simulink model "quad_1_ref_NN_ports_cex"  (R2018b)
settings: Solver=FixedStepAuto  StartTime=0.0  StopTime=20  FixedStep=0.01  RelTol=1e-3
libraries: neural x348, simulink x2
(part 7 of 13)

== system quad_1_ref_NN_ports_cex/nn_1_const/Layer 3/Delays 1 ==
  "p{3}" : Inport  PortDimensions=30
      mask Display: e = 0.06;c1 = [120 230 180]/255;c2 = ([120 230 180]+0)/(256+128);c3 = ([120 230 180]+128)/(256+128);patch([0 1 1 0],[0 0 1 1],c1);patch([0 1 1 1-e 1-e 0+e],[0 0 1 1-e 0+e 0+e],c2);patch([0 0 1 1-e 0+e 0+e],[0 1 1 1-e 1-e 0+e],c3);plot([0 1 1 0 0],[0 0 1 1 0]);
  mux : Mux  Inputs=1
      mask Display: e = 0.06;c1 = [120 150 230]/255;c2 = ([120 150 230]+0)/383;c3 = ([120 150 230]+128)/383;patch([0 1 1 0],[0 0 1 1],c1);patch([0 1 1 1-e 1-e 0+e],[0 0 1 1-e 0+e 0+e],c2);patch([0 0 1 1-e 0+e 0+e],[0 1 1 1-e 1-e 0+e],c3);plot([0 1 1 0 0],[0 0 1 1 0]);disp('Mux')
  "pd{3,2}" : Outport
      mask Display: e = 0.06;c1 = [120 230 180]/255;c2 = ([120 230 180]+0)/(256+128);c3 = ([120 230 180]+128)/(256+128);patch([0 1 1 0],[0 0 1 1],c1);patch([0 1 1 1-e 1-e 0+e],[0 0 1 1-e 0+e 0+e],c2);patch([0 0 1 1-e 0+e 0+e],[0 1 1 1-e 1-e 0+e],c3);plot([0 1 1 0 0],[0 0 1 1 0]);
  wires:
  "p{3}"/1 -> mux/1
  mux/1 -> "pd{3,2}"/1

== system quad_1_ref_NN_ports_cex/nn_1_const/Layer 3/LW{3,2} ==
  "ad{3,2}" : Inport  PortDimensions=30
      mask Display: e = 0.06;c1 = [120 230 180]/255;c2 = ([120 230 180]+0)/(256+128);c3 = ([120 230 180]+128)/(256+128);patch([0 1 1 0],[0 0 1 1],c1);patch([0 1 1 1-e 1-e 0+e],[0 0 1 1-e 0+e 0+e],c2);patch([0 0 1 1-e 0+e 0+e],[0 1 1 1-e 1-e 0+e],c3);plot([0 1 1 0 0],[0 0 1 1 0]);
  "IW{3,2}(1,:)'" : Constant  Value=[0.327928758624340732641400109059759415686130523681640625;-0.55820440747247535018260577999171800911426544189453125;-0.271204192099869789700505862128920853137969970703125;-0.0557769100753577884432843347894959151744842529296875;-0.32758772482643194745577375215361826121807098388671875;0.0203657576424367860179476252824315452016890048980712890625;0.07347277676480434838168775968370027840137481689453125;-0.1579526322944761196342966513839201070368289947509765625;-0.325542754449849980336040289330412633717060089111328125;-0.2238280397863224580046193068483262322843074798583984375;-0.320888627943421378407862221138202585279941558837890625;-0.1946744660874496213320838933213963173329830169677734375;0.50023714377249006712844447974930517375469207763671875;0.1229991088401860277468102822240325622260570526123046875;0.23866675410597848472349369330913759768009185791015625;-0.108125456895287130887339799301116727292537689208984375;-0.491825485074962320819480510181165300309658050537109375;-0.038901938867322134740778238892744411714375019073486328125;0.1040818180648106772157035493364674039185047149658203125;-0.376891881907984116484300329830148257315158843994140625;0.0994428292402699531837839685977087356150150299072265625;-0.07984307261712157710586978964784066192805767059326171875;-0.50048749643499268469071239451295696198940277099609375;-0.45905895663722462440858862464665435254573822021484375;-0.352625950373064878107243202975951135158538818359375;0.1980733704162148944849519693889305926859378814697265625;0.34322332885967565818674529509735293686389923095703125;0.307778286204612172571870587489684112370014190673828125;0.1738835713025933260578170802546082995831966400146484375;-0.23217221679979294091111796660698018968105316162109375]
      mask Display: e = 0.06;c1 = [120 150 230]/255;c2 = ([120 150 230]+0)/383;c3 = ([120 150 230]+128)/383;patch([0 1 1 0],[0 0 1 1],c1);patch([0 1 1 1-e 1-e 0+e],[0 0 1 1-e 0+e 0+e],c2);patch([0 0 1 1-e 0+e 0+e],[0 1 1 1-e 1-e 0+e],c3);plot([0 1 1 0 0],[0 0 1 1 0]);disp('weights');
  "IW{3,2}(2,:)'" : Constant  Value=[-0.10809198337702830006179510746733285486698150634765625;0.1269626329970421074744280076629365794360637664794921875;-0.04521852435502367317798899648551014252007007598876953125;0.1503614425428999312739364313529222272336483001708984375;-0.34833058785911663601808641033130697906017303466796875;0.27979681620865737290415609095362015068531036376953125;-0.3819593294524763482655771440477110445499420166015625;-0.412433724296779657958467169009963981807231903076171875;0.3315789715870411935583206286537460982799530029296875;-0.05820866646834126079124160924038733355700969696044921875;0.306906948135961477053257340230629779398441314697265625;0.37252585636531143631344775712932460010051727294921875;0.308636286795391512338682105109910480678081512451171875;0.2246537489971980050551536578495870344340801239013671875;-0.319882615763760480565025545729440636932849884033203125;-0.00488583502039973728570121380698765278793871402740478515625;0.150436498090291859153211362354340963065624237060546875;0.345641424157331955679950397097854875028133392333984375;0.2227838823473465013069727547190268523991107940673828125;-0.35474970617276746498447437261347658932209014892578125;-0.161697319640236758520046578269102610647678375244140625;-0.44222403234847507125238053049542941153049468994140625;0.211200082911826181319980832995497621595859527587890625;0.42181878561118490988945950448396615684032440185546875;0.03042048915592758528969596909519168548285961151123046875;-0.1897801641563659769129657206576666794717311859130859375;0.1173103045554617918089235217848909087479114532470703125;-0.39376723264394986045999758061952888965606689453125;-0.3681839900591972192245293626911006867885589599609375;0.24280439564999445334336769519723020493984222412109375]
      mask Display: e = 0.06;c1 = [120 150 230]/255;c2 = ([120 150 230]+0)/383;c3 = ([120 150 230]+128)/383;patch([0 1 1 0],[0 0 1 1],c1);patch([0 1 1 1-e 1-e 0+e],[0 0 1 1-e 0+e 0+e],c2);patch([0 0 1 1-e 0+e 0+e],[0 1 1 1-e 1-e 0+e],c3);plot([0 1 1 0 0],[0 0 1 1 0]);disp('weights');
  "IW{3,2}(3,:)'" : Constant  Value=[-0.09740648016186574664754260766130755655467510223388671875;0.1464692614288338745609507896006107330322265625;0.1236987666034225219480191526599810458719730377197265625;0.2380814753048181575678654553485102951526641845703125;0.2303349187376148854422552858522976748645305633544921875;-0.351436586776914750007705379175604321062564849853515625;-0.355839979865836320005456627768580801784992218017578125;-0.12645189201681328317050656551145948469638824462890625;-0.360175944289336913417542973547824658453464508056640625;-0.44453119511866912016984088040771894156932830810546875;0.193836852370338819095962890060036443173885345458984375;0.17499175809764644373700548385386355221271514892578125;0.34285036708253080472985629967297427356243133544921875;-0.28300354963433915767012649666867218911647796630859375;-0.182825795105293231745946513910894282162189483642578125;0.01097749415561990148082482932068160152994096279144287109375;0.38174355853860764131724181424942798912525177001953125;-0.31918936839138634109502845603856258094310760498046875;-0.37820437326661970889318808985990472137928009033203125;0.395234944564560597424218713058508001267910003662109375;0.462073063934263672525304400551249273121356964111328125;-0.31942243334065911763985923244035802781581878662109375;0.415880057336451447458358643416431732475757598876953125;-0.29086088149263644719866306331823579967021942138671875;0.394363290651797926411603611995815299451351165771484375;0.3847585799648449711440889586810953915119171142578125;-0.319785572536297302281838028648053295910358428955078125;0.4503165790658680833757898653857409954071044921875;-0.2488760245881067867390612491362844593822956085205078125;0.231892196915004900059642523046932183206081390380859375]
      mask Display: e = 0.06;c1 = [120 150 230]/255;c2 = ([120 150 230]+0)/383;c3 = ([120 150 230]+128)/383;patch([0 1 1 0],[0 0 1 1],c1);patch([0 1 1 1-e 1-e 0+e],[0 0 1 1-e 0+e 0+e],c2);patch([0 0 1 1-e 0+e 0+e],[0 1 1 1-e 1-e 0+e],c3);plot([0 1 1 0 0],[0 0 1 1 0]);disp('weights');
  Mux : Mux  Inputs=3
      mask Display: e = 0.06;c1 = [120 150 230]/255;c2 = ([120 150 230]+0)/383;c3 = ([120 150 230]+128)/383;patch([0 1 1 0],[0 0 1 1],c1);patch([0 1 1 1-e 1-e 0+e],[0 0 1 1-e 0+e 0+e],c2);patch([0 0 1 1-e 0+e 0+e],[0 1 1 1-e 1-e 0+e],c3);plot([0 1 1 0 0],[0 0 1 1 0]);disp('Mux');
  dotprod1 : neural/Weight Functions/dotprod
  dotprod2 : neural/Weight Functions/dotprod
  dotprod3 : neural/Weight Functions/dotprod
  "lz{3,2}" : Outport
      mask Display: e = 0.06;c1 = [120 230 180]/255;c2 = ([120 230 180]+0)/(256+128);c3 = ([120 230 180]+128)/(256+128);patch([0 1 1 0],[0 0 1 1],c1);patch([0 1 1 1-e 1-e 0+e],[0 0 1 1-e 0+e 0+e],c2);patch([0 0 1 1-e 0+e 0+e],[0 1 1 1-e 1-e 0+e],c3);plot([0 1 1 0 0],[0 0 1 1 0]);
  wires:
  "IW{3,2}(1,:)'"/1 -> dotprod1/1
  "ad{3,2}"/1 -> dotprod1/2, dotprod2/2, dotprod3/2
  dotprod1/1 -> Mux/1
  "IW{3,2}(2,:)'"/1 -> dotprod2/1
  dotprod2/1 -> Mux/2
  "IW{3,2}(3,:)'"/1 -> dotprod3/1
  dotprod3/1 -> Mux/3
  Mux/1 -> "lz{3,2}"/1

== system quad_1_ref_NN_ports_cex/nn_2/Layer 1/Delays 1 ==
  "p{1}" : Inport  PortDimensions=12
      mask Display: e = 0.06;c1 = [120 230 180]/255;c2 = ([120 230 180]+0)/(256+128);c3 = ([120 230 180]+128)/(256+128);patch([0 1 1 0],[0 0 1 1],c1);patch([0 1 1 1-e 1-e 0+e],[0 0 1 1-e 0+e 0+e],c2);patch([0 0 1 1-e 0+e 0+e],[0 1 1 1-e 1-e 0+e],c3);plot([0 1 1 0 0],[0 0 1 1 0]);
  mux : Mux  Inputs=1
      mask Display: e = 0.06;c1 = [120 150 230]/255;c2 = ([120 150 230]+0)/383;c3 = ([120 150 230]+128)/383;patch([0 1 1 0],[0 0 1 1],c1);patch([0 1 1 1-e 1-e 0+e],[0 0 1 1-e 0+e 0+e],c2);patch([0 0 1 1-e 0+e 0+e],[0 1 1 1-e 1-e 0+e],c3);plot([0 1 1 0 0],[0 0 1 1 0]);disp('Mux')
  "pd{1,1}" : Outport
      mask Display: e = 0.06;c1 = [120 230 180]/255;c2 = ([120 230 180]+0)/(256+128);c3 = ([120 230 180]+128)/(256+128);patch([0 1 1 0],[0 0 1 1],c1);patch([0 1 1 1-e 1-e 0+e],[0 0 1 1-e 0+e 0+e],c2);patch([0 0 1 1-e 0+e 0+e],[0 1 1 1-e 1-e 0+e],c3);plot([0 1 1 0 0],[0 0 1 1 0]);
  wires:
  "p{1}"/1 -> mux/1
  mux/1 -> "pd{1,1}"/1

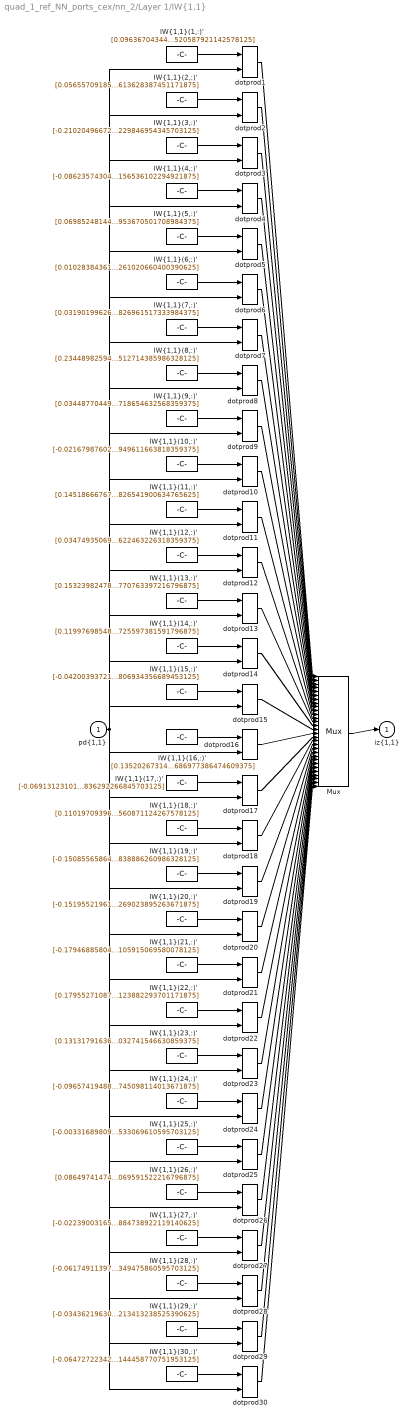
== system quad_1_ref_NN_ports_cex/nn_2/Layer 1/IW{1,1} ==
  "pd{1,1}" : Inport  PortDimensions=12
      mask Display: e = 0.06;c1 = [120 230 180]/255;c2 = ([120 230 180]+0)/(256+128);c3 = ([120 230 180]+128)/(256+128);patch([0 1 1 0],[0 0 1 1],c1);patch([0 1 1 1-e 1-e 0+e],[0 0 1 1-e 0+e 0+e],c2);patch([0 0 1 1-e 0+e 0+e],[0 1 1 1-e 1-e 0+e],c3);plot([0 1 1 0 0],[0 0 1 1 0]);
  "IW{1,1}(1,:)'" : Constant  Value=[0.0963670434492417127270158516694209538400173187255859375;-0.02998489557824503271010740945712313987314701080322265625;0.0198357262796998133624892801663008867762982845306396484375;-0.233494818149912131133305592811666429042816162109375;-0.03964733773014815498836327378739952109754085540771484375;-0.055871328120397911742855967531795613467693328857421875;0.10744492173777138444012990703413379378616809844970703125;-0.0132970271938564719993447482693227357231080532073974609375;0.04911326928811628189652793707864475436508655548095703125;0.03458487107728924758731636757147498428821563720703125;-0.0359117782994806955532141046205651946365833282470703125;0.033230187979102217277205255641092662699520587921142578125]
      mask Display: e = 0.06;c1 = [120 150 230]/255;c2 = ([120 150 230]+0)/383;c3 = ([120 150 230]+128)/383;patch([0 1 1 0],[0 0 1 1],c1);patch([0 1 1 1-e 1-e 0+e],[0 0 1 1-e 0+e 0+e],c2);patch([0 0 1 1-e 0+e 0+e],[0 1 1 1-e 1-e 0+e],c3);plot([0 1 1 0 0],[0 0 1 1 0]);disp('Weights');
  "IW{1,1}(10,:)'" : Constant  Value=[-0.02167987602032135641128007819133927114307880401611328125;0.009575603101159756158633484801612212322652339935302734375;0.06250670535464737664899104174764943309128284454345703125;-0.090538462652213380632559847072116099298000335693359375;0.07271725243563265106416793059906922280788421630859375;-0.0789953395984055728451522782052052207291126251220703125;0.01895637010247945564156424325119587592780590057373046875;-0.02135735691323818741249596087072859518229961395263671875;0.038366841864127775030279821066869772039353847503662109375;0.02384723046277258118319508639615378342568874359130859375;-0.057235972875386113833950929574712063185870647430419921875;0.0258863878959363601095500229121171287260949611663818359375]
      mask Display: e = 0.06;c1 = [120 150 230]/255;c2 = ([120 150 230]+0)/383;c3 = ([120 150 230]+128)/383;patch([0 1 1 0],[0 0 1 1],c1);patch([0 1 1 1-e 1-e 0+e],[0 0 1 1-e 0+e 0+e],c2);patch([0 0 1 1-e 0+e 0+e],[0 1 1 1-e 1-e 0+e],c3);plot([0 1 1 0 0],[0 0 1 1 0]);disp('Weights');
  "IW{1,1}(11,:)'" : Constant  Value=[0.145186667677384750874125529662705957889556884765625;-0.0207530656856331485737854336548480205237865447998046875;-0.066554745131548964653944722158485092222690582275390625;-0.1590044911041626207737209597326000221073627471923828125;-0.0487637284564807760300908512363093905150890350341796875;0.048655868081689403192857668045689933933317661285400390625;0.07936960987217712981678374717375845648348331451416015625;0.0304471844088852160170599603361551999114453792572021484375;0.0237727270256750493337971619212112273089587688446044921875;0.0240198276716949744857831916533541516400873661041259765625;-0.02189528829818498945058991012047044932842254638671875;-0.032706422447001094744312155171428457833826541900634765625]
      mask Display: e = 0.06;c1 = [120 150 230]/255;c2 = ([120 150 230]+0)/383;c3 = ([120 150 230]+128)/383;patch([0 1 1 0],[0 0 1 1],c1);patch([0 1 1 1-e 1-e 0+e],[0 0 1 1-e 0+e 0+e],c2);patch([0 0 1 1-e 0+e 0+e],[0 1 1 1-e 1-e 0+e],c3);plot([0 1 1 0 0],[0 0 1 1 0]);disp('Weights');
  "IW{1,1}(12,:)'" : Constant  Value=[0.034749350696773102786796272312130895443260669708251953125;-0.0736014333872269388425735314740450121462345123291015625;-0.037388165088897341858942269254839629866182804107666015625;0.04756893471249269700340533972848788835108280181884765625;-0.10311435477450504871743675039397203363478183746337890625;0.11262509738201705034033039964924682863056659698486328125;0.0272244869768578333368846955409026122651994228363037109375;-0.018690262067379316557325097392094903625547885894775390625;0.01411732975557855769566106829415730317123234272003173828125;-0.08312468015204542426399569876593886874616146087646484375;-0.052782509266411987980394115993476589210331439971923828125;0.0021418031183407320282297003899429910234175622463226318359375]
      mask Display: e = 0.06;c1 = [120 150 230]/255;c2 = ([120 150 230]+0)/383;c3 = ([120 150 230]+128)/383;patch([0 1 1 0],[0 0 1 1],c1);patch([0 1 1 1-e 1-e 0+e],[0 0 1 1-e 0+e 0+e],c2);patch([0 0 1 1-e 0+e 0+e],[0 1 1 1-e 1-e 0+e],c3);plot([0 1 1 0 0],[0 0 1 1 0]);disp('Weights');
  "IW{1,1}(13,:)'" : Constant  Value=[0.1532398247813539782224978580416063778102397918701171875;0.06953247036407035619465233367009204812347888946533203125;0.00514430221877268216423839675144336069934070110321044921875;-0.171861418147732425421025936884689144790172576904296875;0.046461345556491291663991916038867202587425708770751953125;-0.041708795666123420209370209477128810249269008636474609375;0.041362902434634689352588310384817305020987987518310546875;-0.059449582565483972962372405390851781703531742095947265625;0.0097410876172814020446111271667177788913249969482421875;0.01049776314909686529552867995107590104453265666961669921875;0.033633962417937750266627716655420954339206218719482421875;0.03356606858325654474395349780024844221770763397216796875]
      mask Display: e = 0.06;c1 = [120 150 230]/255;c2 = ([120 150 230]+0)/383;c3 = ([120 150 230]+128)/383;patch([0 1 1 0],[0 0 1 1],c1);patch([0 1 1 1-e 1-e 0+e],[0 0 1 1-e 0+e 0+e],c2);patch([0 0 1 1-e 0+e 0+e],[0 1 1 1-e 1-e 0+e],c3);plot([0 1 1 0 0],[0 0 1 1 0]);disp('Weights');
  "IW{1,1}(14,:)'" : Constant  Value=[0.119976985486957066218138834301498718559741973876953125;0.011074455843699294865789539699107990600168704986572265625;-0.005488285907870558109900027687899637385271489620208740234375;-0.26835186485985718096713981140055693686008453369140625;-0.054938731032241512608482736368387122638523578643798828125;0.0149095357482565936402263417903668596409261226654052734375;0.1518363114705344185662028166916570626199245452880859375;0.027439598095624843920870006286349962465465068817138671875;0.01067608020442331086263809680758640752173960208892822265625;-0.043888814704480368089622999150378745980560779571533203125;0.017947586174126069213929923762407270260155200958251953125;-0.00965387200216295641996833154507839935831725597381591796875]
      mask Display: e = 0.06;c1 = [120 150 230]/255;c2 = ([120 150 230]+0)/383;c3 = ([120 150 230]+128)/383;patch([0 1 1 0],[0 0 1 1],c1);patch([0 1 1 1-e 1-e 0+e],[0 0 1 1-e 0+e 0+e],c2);patch([0 0 1 1-e 0+e 0+e],[0 1 1 1-e 1-e 0+e],c3);plot([0 1 1 0 0],[0 0 1 1 0]);disp('Weights');
  "IW{1,1}(15,:)'" : Constant  Value=[-0.0420039372100648733532324285988579504191875457763671875;-0.002762984426971562719466124491418668185360729694366455078125;0.009128102130523889357061051441633026115596294403076171875;-0.14647320652433093446376233259798027575016021728515625;0.046914158427741624313167534410240477882325649261474609375;-0.0277928987001266648848574192243177094496786594390869140625;-0.054667118131341237152742706939534400589764118194580078125;-0.0251059154922964877787450177493155933916568756103515625;-0.07223823520848195178789552528542117215692996978759765625;-0.0167336904534491660856421191283516236580908298492431640625;0.04191004740064542544164538639961392618715763092041015625;-0.051084165943738442383637021748654660768806934356689453125]
      mask Display: e = 0.06;c1 = [120 150 230]/255;c2 = ([120 150 230]+0)/383;c3 = ([120 150 230]+128)/383;patch([0 1 1 0],[0 0 1 1],c1);patch([0 1 1 1-e 1-e 0+e],[0 0 1 1-e 0+e 0+e],c2);patch([0 0 1 1-e 0+e 0+e],[0 1 1 1-e 1-e 0+e],c3);plot([0 1 1 0 0],[0 0 1 1 0]);disp('Weights');
  "IW{1,1}(16,:)'" : Constant  Value=[0.1352026731469619935666059973300434648990631103515625;-0.047386257163045071572060606968079810030758380889892578125;-0.041907967250772427958427357452819705940783023834228515625;-0.1563236402964026383610729453721432946622371673583984375;-0.0235850694502852016587457484320111689157783985137939453125;0.0116247438816773455971809170250708120875060558319091796875;-0.040658251599097562645201975328745902515947818756103515625;0.05251236963362911069896910021270741708576679229736328125;-0.01102946874268842698818549052930393372662365436553955078125;-0.005492271286121085116516127300201333127915859222412109375;0.0234165142870034724553729432727777748368680477142333984375;-0.040401643285461863452923125805682502686977386474609375]
      mask Display: e = 0.06;c1 = [120 150 230]/255;c2 = ([120 150 230]+0)/383;c3 = ([120 150 230]+128)/383;patch([0 1 1 0],[0 0 1 1],c1);patch([0 1 1 1-e 1-e 0+e],[0 0 1 1-e 0+e 0+e],c2);patch([0 0 1 1-e 0+e 0+e],[0 1 1 1-e 1-e 0+e],c3);plot([0 1 1 0 0],[0 0 1 1 0]);disp('Weights');
  "IW{1,1}(17,:)'" : Constant  Value=[-0.06913123101193986708157268594732158817350864410400390625;-0.042455432406210295848136837548736366443336009979248046875;0.01369205857005208193388767767828539945185184478759765625;0.11383782048737491054968273829217650927603244781494140625;-0.060466490543143340541387686926100286655128002166748046875;0.0188919876523014375335751680040630162693560123443603515625;-0.048107408169124142582884218199978931806981563568115234375;-0.01528739302378535717952257044771613436751067638397216796875;-0.05144260921280367770958008577508735470473766326904296875;-0.05096443422523273814039868057079729624092578887939453125;-0.02945636339152606086866370560528594069182872772216796875;-0.0171135307590550740652890482351722312159836292266845703125]
      mask Display: e = 0.06;c1 = [120 150 230]/255;c2 = ([120 150 230]+0)/383;c3 = ([120 150 230]+128)/383;patch([0 1 1 0],[0 0 1 1],c1);patch([0 1 1 1-e 1-e 0+e],[0 0 1 1-e 0+e 0+e],c2);patch([0 0 1 1-e 0+e 0+e],[0 1 1 1-e 1-e 0+e],c3);plot([0 1 1 0 0],[0 0 1 1 0]);disp('Weights');
  "IW{1,1}(18,:)'" : Constant  Value=[0.11019709396075240415147078465452068485319614410400390625;0.04926979088195641842684580069544608704745769500732421875;-0.04838283233660277404819538560332148335874080657958984375;-0.00963057704813059800574848168253083713352680206298828125;-0.009613748734012779462165809718499076552689075469970703125;-0.0325377541810061010618682075801189057528972625732421875;0.036575137550091195437484969943398027680814266204833984375;-0.01572076232144341279006738432144629769027233123779296875;-0.0076129085484086013446702878582073026336729526519775390625;-0.025254150868068779567376935801803483627736568450927734375;-0.046262519846408341195331814788005431182682514190673828125;-0.040657774038491974188946898038921062834560871124267578125]
      mask Display: e = 0.06;c1 = [120 150 230]/255;c2 = ([120 150 230]+0)/383;c3 = ([120 150 230]+128)/383;patch([0 1 1 0],[0 0 1 1],c1);patch([0 1 1 1-e 1-e 0+e],[0 0 1 1-e 0+e 0+e],c2);patch([0 0 1 1-e 0+e 0+e],[0 1 1 1-e 1-e 0+e],c3);plot([0 1 1 0 0],[0 0 1 1 0]);disp('Weights');
  "IW{1,1}(19,:)'" : Constant  Value=[-0.1508556586474403271580513319349847733974456787109375;-0.018213648918746681848457313890321529470384120941162109375;-0.027881145100316861995537465190864168107509613037109375;0.1829520964826169826533686091352137736976146697998046875;-0.048285945392414646171186376477635349147021770477294921875;0.054448955430182501002978057158543379046022891998291015625;-0.10379420330937040584107222684906446374952793121337890625;0.019158116711153423683544616551444050855934619903564453125;0.039685064615922575892437151878766599111258983612060546875;-0.0231794568681364422657598112209598184563219547271728515625;0.0055987528789933523054589414869042229838669300079345703125;-0.016475006097132767479696013879220117814838886260986328125]
      mask Display: e = 0.06;c1 = [120 150 230]/255;c2 = ([120 150 230]+0)/383;c3 = ([120 150 230]+128)/383;patch([0 1 1 0],[0 0 1 1],c1);patch([0 1 1 1-e 1-e 0+e],[0 0 1 1-e 0+e 0+e],c2);patch([0 0 1 1-e 0+e 0+e],[0 1 1 1-e 1-e 0+e],c3);plot([0 1 1 0 0],[0 0 1 1 0]);disp('Weights');
  "IW{1,1}(2,:)'" : Constant  Value=[0.0565570918586223714275007523610838688910007476806640625;-0.04556319233391274703404150159258279018104076385498046875;-0.00525403129053085560240532458919915370643138885498046875;-0.02284769747955449348264522768658935092389583587646484375;-0.043835671970937857555572492174178478308022022247314453125;-0.041265694783639894627214061983977444469928741455078125;-0.0137285514204576741814634033289621584117412567138671875;0.0251722865985351089423982529069689917378127574920654296875;0.041086109140649702820002886483052861876785755157470703125;0.044350373424499579810831306758700520731508731842041015625;0.0297244917886227318082337234272927162237465381622314453125;-0.017723255711821921110082911354766110889613628387451171875]
      mask Display: e = 0.06;c1 = [120 150 230]/255;c2 = ([120 150 230]+0)/383;c3 = ([120 150 230]+128)/383;patch([0 1 1 0],[0 0 1 1],c1);patch([0 1 1 1-e 1-e 0+e],[0 0 1 1-e 0+e 0+e],c2);patch([0 0 1 1-e 0+e 0+e],[0 1 1 1-e 1-e 0+e],c3);plot([0 1 1 0 0],[0 0 1 1 0]);disp('Weights');
  "IW{1,1}(20,:)'" : Constant  Value=[-0.151955219615692527224126706641982309520244598388671875;-0.00644169278533961685295761157021843246184289455413818359375;-0.0014910754802380308918496876202652856591157615184783935546875;0.2178704362857331877645350459715700708329677581787109375;-0.0159318550347393970978426835927166393958032131195068359375;-0.0306780730434982780441277583349801716394722461700439453125;-0.165514568504929793224533796092146076261997222900390625;-0.03816639102354042745179896201079827733337879180908203125;0.048144549460101222770891382651825551874935626983642578125;-0.04926366893596752227768575949085061438381671905517578125;0.00583623873334166744231144008381306775845587253570556640625;-0.038415089615007107226585247872208128683269023895263671875]
      mask Display: e = 0.06;c1 = [120 150 230]/255;c2 = ([120 150 230]+0)/383;c3 = ([120 150 230]+128)/383;patch([0 1 1 0],[0 0 1 1],c1);patch([0 1 1 1-e 1-e 0+e],[0 0 1 1-e 0+e 0+e],c2);patch([0 0 1 1-e 0+e 0+e],[0 1 1 1-e 1-e 0+e],c3);plot([0 1 1 0 0],[0 0 1 1 0]);disp('Weights');
  "IW{1,1}(21,:)'" : Constant  Value=[-0.1794688580443983827450438184314407408237457275390625;-0.028516979645142041810412791846829350106418132781982421875;-0.0090720363478705122461942522704703151248395442962646484375;0.1255159624610372726127849318800144828855991363525390625;-0.039600857039564930917041607472128816880285739898681640625;-0.032308661764052060139107425129623152315616607666015625;-0.016981166020414890927003881415657815523445606231689453125;0.03632720422941571047914521841448731720447540283203125;-0.000448192583532860087947025107268927968107163906097412109375;0.01167939131266501097405896558711901889182627201080322265625;0.054971223698895892162408216563562746159732341766357421875;0.0015702044461439715501704927902437702869065105915069580078125]
      mask Display: e = 0.06;c1 = [120 150 230]/255;c2 = ([120 150 230]+0)/383;c3 = ([120 150 230]+128)/383;patch([0 1 1 0],[0 0 1 1],c1);patch([0 1 1 1-e 1-e 0+e],[0 0 1 1-e 0+e 0+e],c2);patch([0 0 1 1-e 0+e 0+e],[0 1 1 1-e 1-e 0+e],c3);plot([0 1 1 0 0],[0 0 1 1 0]);disp('Weights');
  "IW{1,1}(22,:)'" : Constant  Value=[0.179552710875321486216904531829641200602054595947265625;-0.0271027099443047377047566470764650148339569568634033203125;-0.0668122147617648820538960308113018982112407684326171875;-0.2312456882295024496176694128735107369720935821533203125;-0.0572558162532104952813227782826288603246212005615234375;0.092657437825664545893999957115738652646541595458984375;0.10313999906360561686913257517517195083200931549072265625;-0.0271104480045279705446858997675008140504360198974609375;0.0114841311289845850185376008312232443131506443023681640625;0.030408296426441328019762977419304661452770233154296875;0.0307288869733456648791758425431908108294010162353515625;-0.017814450901100280233446682132125715725123882293701171875]
      mask Display: e = 0.06;c1 = [120 150 230]/255;c2 = ([120 150 230]+0)/383;c3 = ([120 150 230]+128)/383;patch([0 1 1 0],[0 0 1 1],c1);patch([0 1 1 1-e 1-e 0+e],[0 0 1 1-e 0+e 0+e],c2);patch([0 0 1 1-e 0+e 0+e],[0 1 1 1-e 1-e 0+e],c3);plot([0 1 1 0 0],[0 0 1 1 0]);disp('Weights');
  "IW{1,1}(23,:)'" : Constant  Value=[0.13131791636346878959784589824266731739044189453125;0.0193863240459271994609036227075193892233073711395263671875;0.00715174559120907750442430739212795742787420749664306640625;0.05486655159595266173511163287912495434284210205078125;0.0401442208550966406210847026159171946346759796142578125;0.04377915024574856317496340807338128797709941864013671875;-0.031675194504130137207464912307841586880385875701904296875;0.01981077134609214585037051392646390013396739959716796875;-0.00963765867608215066886234723142479197122156620025634765625;-0.047466276118460902500029163775252527557313442230224609375;-0.01166577285425598499435384525213521555997431278228759765625;-0.0197833266932704032736722865593037568032741546630859375]
      mask Display: e = 0.06;c1 = [120 150 230]/255;c2 = ([120 150 230]+0)/383;c3 = ([120 150 230]+128)/383;patch([0 1 1 0],[0 0 1 1],c1);patch([0 1 1 1-e 1-e 0+e],[0 0 1 1-e 0+e 0+e],c2);patch([0 0 1 1-e 0+e 0+e],[0 1 1 1-e 1-e 0+e],c3);plot([0 1 1 0 0],[0 0 1 1 0]);disp('Weights');
  "IW{1,1}(24,:)'" : Constant  Value=[-0.09657419488549467967430928183603100478649139404296875;0.0241557095740239750891742431804232182912528514862060546875;0.047777796487195108021683864762962912209331989288330078125;0.1623879706509529785574130755776423029601573944091796875;-0.0456818379862133083779696107740164734423160552978515625;-0.0200364773549174639277747900223403121344745159149169921875;-0.07744412917817887487270667179473093710839748382568359375;0.020062417659231446265266640693880617618560791015625;-0.061868560782029576039509066731625352986156940460205078125;0.067823465106819968983842272791662253439426422119140625;0.03182642212306575901781258153278031386435031890869140625;0.031288377204634225392521074127216706983745098114013671875]
      mask Display: e = 0.06;c1 = [120 150 230]/255;c2 = ([120 150 230]+0)/383;c3 = ([120 150 230]+128)/383;patch([0 1 1 0],[0 0 1 1],c1);patch([0 1 1 1-e 1-e 0+e],[0 0 1 1-e 0+e 0+e],c2);patch([0 0 1 1-e 0+e 0+e],[0 1 1 1-e 1-e 0+e],c3);plot([0 1 1 0 0],[0 0 1 1 0]);disp('Weights');
  "IW{1,1}(25,:)'" : Constant  Value=[-0.00331689809484806384654032029857262386940419673919677734375;-0.000282766784016928360810660958435391876264475286006927490234375;0.00831186986145609520149069027183941216208040714263916015625;-0.030673501351737054998469744759859167970716953277587890625;-0.043560595315479601341568383077174075879156589508056640625;-0.059214945748563764527094832601505913771688938140869140625;-0.0073905937341639908744195253120778943412005901336669921875;0.051288395431760676335120052726779249496757984161376953125;0.07664423673696525718401773019650136120617389678955078125;0.03814554995943862658602796500417753122746944427490234375;-0.01543352955019334192543478678771862178109586238861083984375;-0.01042068425015845074821374538487361860461533069610595703125]
      mask Display: e = 0.06;c1 = [120 150 230]/255;c2 = ([120 150 230]+0)/383;c3 = ([120 150 230]+128)/383;patch([0 1 1 0],[0 0 1 1],c1);patch([0 1 1 1-e 1-e 0+e],[0 0 1 1-e 0+e 0+e],c2);patch([0 0 1 1-e 0+e 0+e],[0 1 1 1-e 1-e 0+e],c3);plot([0 1 1 0 0],[0 0 1 1 0]);disp('Weights');
  "IW{1,1}(26,:)'" : Constant  Value=[0.0864974147458101028096422169255674816668033599853515625;0.040666463190978892339177974690755945630371570587158203125;0.00946664496001405585123844588224528706632554531097412109375;-0.04383941989612703815648586669340147636830806732177734375;0.03127239447551567741445666115396306850016117095947265625;-0.0157148210500004971434950817865683347918093204498291015625;0.04288729634681824609554467997440951876342296600341796875;0.045272834343532318557290494709377526305615901947021484375;0.002130217585906197912126724958170598256401717662811279296875;-0.039506203531120311078783657876556389965116977691650390625;-0.04856855204270905945751479748651036061346530914306640625;-0.026968614233296654691951488302947836928069591522216796875]
      mask Display: e = 0.06;c1 = [120 150 230]/255;c2 = ([120 150 230]+0)/383;c3 = ([120 150 230]+128)/383;patch([0 1 1 0],[0 0 1 1],c1);patch([0 1 1 1-e 1-e 0+e],[0 0 1 1-e 0+e 0+e],c2);patch([0 0 1 1-e 0+e 0+e],[0 1 1 1-e 1-e 0+e],c3);plot([0 1 1 0 0],[0 0 1 1 0]);disp('Weights');
  "IW{1,1}(27,:)'" : Constant  Value=[-0.02239003165257756611250528067103005014359951019287109375;-0.0538707440898208156365711829494102858006954193115234375;-0.0330754878358191783949138198295258916914463043212890625;-0.035570346482772803586858145763471839018166065216064453125;0.02574992367182293850902397025492973625659942626953125;-0.058123079327492187251547051118905073963105678558349609375;0.060044248722781239091528249218754353933036327362060546875;0.007465947049040411176434872686513699591159820556640625;0.01239835981269137889226872317749439389444887638092041015625;0.0094665618527167323670301612992261652834713459014892578125;0.0226138083092675967744611398302367888391017913818359375;-0.0659262781382616014358433176312246359884738922119140625]
      mask Display: e = 0.06;c1 = [120 150 230]/255;c2 = ([120 150 230]+0)/383;c3 = ([120 150 230]+128)/383;patch([0 1 1 0],[0 0 1 1],c1);patch([0 1 1 1-e 1-e 0+e],[0 0 1 1-e 0+e 0+e],c2);patch([0 0 1 1-e 0+e 0+e],[0 1 1 1-e 1-e 0+e],c3);plot([0 1 1 0 0],[0 0 1 1 0]);disp('Weights');
  "IW{1,1}(28,:)'" : Constant  Value=[-0.06174911397351805220079512537267873995006084442138671875;-0.02906210355952566770643130666940123774111270904541015625;0.034023060196417896638987343749249703250825405120849609375;0.023048831489107919623382514373588492162525653839111328125;0.01865692732944046472454147078678943216800689697265625;0.0311337387192645136113622328366545843891799449920654296875;0.039489979733197101696706710072248824872076511383056640625;0.0267679752780296924263847557767803664319217205047607421875;0.0530894458170886041070701821809052489697933197021484375;-0.046325994620529387102436658096848987042903900146484375;0.02601931784012596893251867413709987886250019073486328125;0.022959347382819468574854937514828634448349475860595703125]
      mask Display: e = 0.06;c1 = [120 150 230]/255;c2 = ([120 150 230]+0)/383;c3 = ([120 150 230]+128)/383;patch([0 1 1 0],[0 0 1 1],c1);patch([0 1 1 1-e 1-e 0+e],[0 0 1 1-e 0+e 0+e],c2);patch([0 0 1 1-e 0+e 0+e],[0 1 1 1-e 1-e 0+e],c3);plot([0 1 1 0 0],[0 0 1 1 0]);disp('Weights');
  "IW{1,1}(29,:)'" : Constant  Value=[-0.034362196308690327872792380503597087226808071136474609375;0.047802343289393804670606158424561726860702037811279296875;-0.043941192910080535682926239360313047654926776885986328125;0.00884490236447522427953860102434191503562033176422119140625;-0.0384940746721876558833486114963307045400142669677734375;-0.0292364023388453873886216882738153799436986446380615234375;0.040054045736892841811371823723675333894789218902587890625;0.02839082147759265650766025146367610432207584381103515625;0.0276409810466857717992095189174506231211125850677490234375;0.049653817107354066007207649136034888215363025665283203125;-0.018556535309921622090012505168488132767379283905029296875;-0.0042383709736225939901377302021501236595213413238525390625]
      mask Display: e = 0.06;c1 = [120 150 230]/255;c2 = ([120 150 230]+0)/383;c3 = ([120 150 230]+128)/383;patch([0 1 1 0],[0 0 1 1],c1);patch([0 1 1 1-e 1-e 0+e],[0 0 1 1-e 0+e 0+e],c2);patch([0 0 1 1-e 0+e 0+e],[0 1 1 1-e 1-e 0+e],c3);plot([0 1 1 0 0],[0 0 1 1 0]);disp('Weights');
  "IW{1,1}(3,:)'" : Constant  Value=[-0.2102049667287736733900516128414892591536045074462890625;0.05377313104783233710382006620420725084841251373291015625;0.0148167836257803477162386940335636609233915805816650390625;0.1618907253628284192981112710185698233544826507568359375;0.0280826467808530273739808791333416593261063098907470703125;0.036311406062564145769133716612486750818789005279541015625;-0.062374123493120110783838327961348113603889942169189453125;0.03197512392109873313739143441125634126365184783935546875;-0.00723855197664829801140751186494526336900889873504638671875;-0.0014061660318630576915754915034995065070688724517822265625;-0.03206732177008009276875100113102234899997711181640625;-0.01103754683288076139657807317462356877513229846954345703125]
      mask Display: e = 0.06;c1 = [120 150 230]/255;c2 = ([120 150 230]+0)/383;c3 = ([120 150 230]+128)/383;patch([0 1 1 0],[0 0 1 1],c1);patch([0 1 1 1-e 1-e 0+e],[0 0 1 1-e 0+e 0+e],c2);patch([0 0 1 1-e 0+e 0+e],[0 1 1 1-e 1-e 0+e],c3);plot([0 1 1 0 0],[0 0 1 1 0]);disp('Weights');
  "IW{1,1}(30,:)'" : Constant  Value=[-0.0647272234224625930831820141975185833871364593505859375;-0.00103525983680078184114015105166117791668511927127838134765625;-0.04603733823568430250094962730145198293030261993408203125;0.033532641206834308544859624134915065951645374298095703125;0.010792696704966464604780185254639945924282073974609375;-0.037358503116967832491379652992691262625157833099365234375;0.037127815083188020484072922045015729963779449462890625;-0.0174011380525709476174700540695994277484714984893798828125;0.0243385492782321084803687227804402937181293964385986328125;0.04283103501804554069654074055506498552858829498291015625;-0.05571776036524682396144925178305129520595073699951171875;-0.025143638744761720449361064311233349144458770751953125]
      mask Display: e = 0.06;c1 = [120 150 230]/255;c2 = ([120 150 230]+0)/383;c3 = ([120 150 230]+128)/383;patch([0 1 1 0],[0 0 1 1],c1);patch([0 1 1 1-e 1-e 0+e],[0 0 1 1-e 0+e 0+e],c2);patch([0 0 1 1-e 0+e 0+e],[0 1 1 1-e 1-e 0+e],c3);plot([0 1 1 0 0],[0 0 1 1 0]);disp('Weights');
  "IW{1,1}(4,:)'" : Constant  Value=[-0.086235743041017276500070920519647188484668731689453125;-0.0149966577015172193576564296790820662863552570343017578125;-0.031564764179194092219571388113763532601296901702880859375;0.09766885054489993223114652209915220737457275390625;0.0217664819637368445182090681555564515292644500732421875;-0.031555428724406454910056396556683466769754886627197265625;-0.0298792461028349991269958962902819621376693248748779296875;-0.025119472963766160955589867853632313199341297149658203125;-0.0118177061221431643767143526702056988142430782318115234375;-0.035573933545714371551316190789293614216148853302001953125;0.052553496804224560101648222598669235594570636749267578125;-0.010976038270683552422468665099586360156536102294921875]
      mask Display: e = 0.06;c1 = [120 150 230]/255;c2 = ([120 150 230]+0)/383;c3 = ([120 150 230]+128)/383;patch([0 1 1 0],[0 0 1 1],c1);patch([0 1 1 1-e 1-e 0+e],[0 0 1 1-e 0+e 0+e],c2);patch([0 0 1 1-e 0+e 0+e],[0 1 1 1-e 1-e 0+e],c3);plot([0 1 1 0 0],[0 0 1 1 0]);disp('Weights');
  "IW{1,1}(5,:)'" : Constant  Value=[0.06985248144510837475795739237582893110811710357666015625;-0.0307486201456255194008893028012607828713953495025634765625;0.02894376433176391871793242671628831885755062103271484375;-0.005346327416415806894900430989991946262307465076446533203125;0.01188390260536431770888032843913606484420597553253173828125;-0.0114613562961506480764040105668755131773650646209716796875;0.04236187567373904394596451083998545072972774505615234375;0.06718769680293833201911724017918459139764308929443359375;0.06466020183756408801212245407441514544188976287841796875;-0.0220039215718493587348181250717971124686300754547119140625;-0.039260518366975138970786929348832927644252777099609375;-0.00105389130048585250541692825976269887178204953670501708984375]
      mask Display: e = 0.06;c1 = [120 150 230]/255;c2 = ([120 150 230]+0)/383;c3 = ([120 150 230]+128)/383;patch([0 1 1 0],[0 0 1 1],c1);patch([0 1 1 1-e 1-e 0+e],[0 0 1 1-e 0+e 0+e],c2);patch([0 0 1 1-e 0+e 0+e],[0 1 1 1-e 1-e 0+e],c3);plot([0 1 1 0 0],[0 0 1 1 0]);disp('Weights');
  "IW{1,1}(6,:)'" : Constant  Value=[0.01028384361434746437080622882831448805518448352813720703125;0.044526993659847739770452079710594261996448040008544921875;-0.040360747663441519372806709498036070726811885833740234375;0.0728533726619254584644380656754947267472743988037109375;0.042600037093803895527077685301264864392578601837158203125;-0.010512535420402986663379607534807291813194751739501953125;-0.030739757003768373999630370008162572048604488372802734375;-0.029063052721925976273897873625173815526068210601806640625;0.03735417973416042813905590946887969039380550384521484375;0.0084287830330014683333228475703435833565890789031982421875;-0.0040596027592133578087985057436526403762400150299072265625;0.01529846722711373542546997583713164203800261020660400390625]
      mask Display: e = 0.06;c1 = [120 150 230]/255;c2 = ([120 150 230]+0)/383;c3 = ([120 150 230]+128)/383;patch([0 1 1 0],[0 0 1 1],c1);patch([0 1 1 1-e 1-e 0+e],[0 0 1 1-e 0+e 0+e],c2);patch([0 0 1 1-e 0+e 0+e],[0 1 1 1-e 1-e 0+e],c3);plot([0 1 1 0 0],[0 0 1 1 0]);disp('Weights');
  "IW{1,1}(7,:)'" : Constant  Value=[0.031901996267111536187410791853835689835250377655029296875;0.025743864317476737590961732848882093094289302825927734375;0.01263784780899015157407117015964104211889207363128662109375;-0.07141648945085062039073164896763046272099018096923828125;0.027735381692866767355809543005307205021381378173828125;0.0226746721237255748071515171204737271182239055633544921875;0.03605581098147207785853396444508689455687999725341796875;0.063932001500569823893016518923104740679264068603515625;0.0687963867839390952330091977273696102201938629150390625;0.004194467822440259459348954607094128732569515705108642578125;-0.03837213298740198286207458977514761500060558319091796875;-0.00893313762727549441622354464698219089768826961517333984375]
      mask Display: e = 0.06;c1 = [120 150 230]/255;c2 = ([120 150 230]+0)/383;c3 = ([120 150 230]+128)/383;patch([0 1 1 0],[0 0 1 1],c1);patch([0 1 1 1-e 1-e 0+e],[0 0 1 1-e 0+e 0+e],c2);patch([0 0 1 1-e 0+e 0+e],[0 1 1 1-e 1-e 0+e],c3);plot([0 1 1 0 0],[0 0 1 1 0]);disp('Weights');
  "IW{1,1}(8,:)'" : Constant  Value=[0.23448982594603406948152723998646251857280731201171875;-0.01130592823405165113503922924564903951250016689300537109375;0.067290545698162229637517839364591054618358612060546875;-0.2044532018384969951352303496605600230395793914794921875;0.017557456415888690604010236029353109188377857208251953125;-0.039901636777410744161276312524933018721640110015869140625;0.204354741339915768616464220031048171222209930419921875;-0.04894889606208895072025910621960065327584743499755859375;-0.02592801255776676361275434601338929496705532073974609375;0.0030432187082790542083376994497712075826711952686309814453125;0.0409640248584569321987913781413226388394832611083984375;-0.017625613893270615506470022637586225755512714385986328125]
      mask Display: e = 0.06;c1 = [120 150 230]/255;c2 = ([120 150 230]+0)/383;c3 = ([120 150 230]+128)/383;patch([0 1 1 0],[0 0 1 1],c1);patch([0 1 1 1-e 1-e 0+e],[0 0 1 1-e 0+e 0+e],c2);patch([0 0 1 1-e 0+e 0+e],[0 1 1 1-e 1-e 0+e],c3);plot([0 1 1 0 0],[0 0 1 1 0]);disp('Weights');
  "IW{1,1}(9,:)'" : Constant  Value=[0.03448770449633757617657892069473746232688426971435546875;-0.03858613201594847386122211219117161817848682403564453125;-0.0028984332577655269776173430074095449526794254779815673828125;0.114804812734617567304695739949238486588001251220703125;0.00850861193611015566296007506252863095141947269439697265625;-0.0195065463125524314602632358628397923894226551055908203125;-0.0679665398584372304480183402120019309222698211669921875;0.005850141405491567081487147561347228474915027618408203125;0.0008432308526460214302689077925379024236463010311126708984375;0.0164759783491125154364365101855582906864583492279052734375;-0.0564263332476396539671981145147583447396755218505859375;0.023866500179500226008766361474044970236718654632568359375]
      mask Display: e = 0.06;c1 = [120 150 230]/255;c2 = ([120 150 230]+0)/383;c3 = ([120 150 230]+128)/383;patch([0 1 1 0],[0 0 1 1],c1);patch([0 1 1 1-e 1-e 0+e],[0 0 1 1-e 0+e 0+e],c2);patch([0 0 1 1-e 0+e 0+e],[0 1 1 1-e 1-e 0+e],c3);plot([0 1 1 0 0],[0 0 1 1 0]);disp('Weights');
  Mux : Mux  Inputs=30
      mask Display: e = 0.06;c1 = [120 150 230]/255;c2 = ([120 150 230]+0)/383;c3 = ([120 150 230]+128)/383;patch([0 1 1 0],[0 0 1 1],c1);patch([0 1 1 1-e 1-e 0+e],[0 0 1 1-e 0+e 0+e],c2);patch([0 0 1 1-e 0+e 0+e],[0 1 1 1-e 1-e 0+e],c3);plot([0 1 1 0 0],[0 0 1 1 0]);disp('Mux');
  dotprod{1..30} (30 alike) : neural/Weight Functions/dotprod
  "iz{1,1}" : Outport
      mask Display: e = 0.06;c1 = [120 230 180]/255;c2 = ([120 230 180]+0)/(256+128);c3 = ([120 230 180]+128)/(256+128);patch([0 1 1 0],[0 0 1 1],c1);patch([0 1 1 1-e 1-e 0+e],[0 0 1 1-e 0+e 0+e],c2);patch([0 0 1 1-e 0+e 0+e],[0 1 1 1-e 1-e 0+e],c3);plot([0 1 1 0 0],[0 0 1 1 0]);
  wires:
  "IW{1,1}(1,:)'"/1 -> dotprod1/1
  "pd{1,1}"/1 -> dotprod1/2, dotprod2/2, dotprod3/2, dotprod4/2, dotprod5/2, dotprod6/2, dotprod7/2, dotprod8/2, dotprod9/2, dotprod10/2, dotprod11/2, dotprod12/2, dotprod13/2, dotprod14/2, dotprod15/2, dotprod16/2, dotprod17/2, dotprod18/2, dotprod19/2, dotprod20/2, dotprod21/2, dotprod22/2, dotprod23/2, dotprod24/2, dotprod25/2, dotprod26/2, dotprod27/2, dotprod28/2, dotprod29/2, dotprod30/2
  dotprod1/1 -> Mux/1
  "IW{1,1}(2,:)'"/1 -> dotprod2/1
  dotprod2/1 -> Mux/2
  "IW{1,1}(3,:)'"/1 -> dotprod3/1
  dotprod3/1 -> Mux/3
  "IW{1,1}(4,:)'"/1 -> dotprod4/1
  dotprod4/1 -> Mux/4
  "IW{1,1}(5,:)'"/1 -> dotprod5/1
  dotprod5/1 -> Mux/5
  "IW{1,1}(6,:)'"/1 -> dotprod6/1
  dotprod6/1 -> Mux/6
  "IW{1,1}(7,:)'"/1 -> dotprod7/1
  dotprod7/1 -> Mux/7
  "IW{1,1}(8,:)'"/1 -> dotprod8/1
  dotprod8/1 -> Mux/8
  "IW{1,1}(9,:)'"/1 -> dotprod9/1
  dotprod9/1 -> Mux/9
  "IW{1,1}(10,:)'"/1 -> dotprod10/1
  dotprod10/1 -> Mux/10
  "IW{1,1}(11,:)'"/1 -> dotprod11/1
  dotprod11/1 -> Mux/11
  "IW{1,1}(12,:)'"/1 -> dotprod12/1
  dotprod12/1 -> Mux/12
  "IW{1,1}(13,:)'"/1 -> dotprod13/1
  dotprod13/1 -> Mux/13
  "IW{1,1}(14,:)'"/1 -> dotprod14/1
  dotprod14/1 -> Mux/14
  "IW{1,1}(15,:)'"/1 -> dotprod15/1
  dotprod15/1 -> Mux/15
  "IW{1,1}(16,:)'"/1 -> dotprod16/1
  dotprod16/1 -> Mux/16
  "IW{1,1}(17,:)'"/1 -> dotprod17/1
  dotprod17/1 -> Mux/17
  "IW{1,1}(18,:)'"/1 -> dotprod18/1
  dotprod18/1 -> Mux/18
  "IW{1,1}(19,:)'"/1 -> dotprod19/1
  dotprod19/1 -> Mux/19
  "IW{1,1}(20,:)'"/1 -> dotprod20/1
  dotprod20/1 -> Mux/20
  "IW{1,1}(21,:)'"/1 -> dotprod21/1
  dotprod21/1 -> Mux/21
  "IW{1,1}(22,:)'"/1 -> dotprod22/1
  dotprod22/1 -> Mux/22
  "IW{1,1}(23,:)'"/1 -> dotprod23/1
  dotprod23/1 -> Mux/23
  "IW{1,1}(24,:)'"/1 -> dotprod24/1
  dotprod24/1 -> Mux/24
  "IW{1,1}(25,:)'"/1 -> dotprod25/1
  dotprod25/1 -> Mux/25
  "IW{1,1}(26,:)'"/1 -> dotprod26/1
  dotprod26/1 -> Mux/26
  "IW{1,1}(27,:)'"/1 -> dotprod27/1
  dotprod27/1 -> Mux/27
  "IW{1,1}(28,:)'"/1 -> dotprod28/1
  dotprod28/1 -> Mux/28
  "IW{1,1}(29,:)'"/1 -> dotprod29/1
  dotprod29/1 -> Mux/29
  "IW{1,1}(30,:)'"/1 -> dotprod30/1
  dotprod30/1 -> Mux/30
  Mux/1 -> "iz{1,1}"/1

== system quad_1_ref_NN_ports_cex/nn_2/Layer 2/Delays 1 ==
  "p{2}" : Inport  PortDimensions=30
      mask Display: e = 0.06;c1 = [120 230 180]/255;c2 = ([120 230 180]+0)/(256+128);c3 = ([120 230 180]+128)/(256+128);patch([0 1 1 0],[0 0 1 1],c1);patch([0 1 1 1-e 1-e 0+e],[0 0 1 1-e 0+e 0+e],c2);patch([0 0 1 1-e 0+e 0+e],[0 1 1 1-e 1-e 0+e],c3);plot([0 1 1 0 0],[0 0 1 1 0]);
  mux : Mux  Inputs=1
      mask Display: e = 0.06;c1 = [120 150 230]/255;c2 = ([120 150 230]+0)/383;c3 = ([120 150 230]+128)/383;patch([0 1 1 0],[0 0 1 1],c1);patch([0 1 1 1-e 1-e 0+e],[0 0 1 1-e 0+e 0+e],c2);patch([0 0 1 1-e 0+e 0+e],[0 1 1 1-e 1-e 0+e],c3);plot([0 1 1 0 0],[0 0 1 1 0]);disp('Mux')
  "pd{2,1}" : Outport
      mask Display: e = 0.06;c1 = [120 230 180]/255;c2 = ([120 230 180]+0)/(256+128);c3 = ([120 230 180]+128)/(256+128);patch([0 1 1 0],[0 0 1 1],c1);patch([0 1 1 1-e 1-e 0+e],[0 0 1 1-e 0+e 0+e],c2);patch([0 0 1 1-e 0+e 0+e],[0 1 1 1-e 1-e 0+e],c3);plot([0 1 1 0 0],[0 0 1 1 0]);
  wires:
  "p{2}"/1 -> mux/1
  mux/1 -> "pd{2,1}"/1
